simulink model "watertankLSTM"  (R2026a)
settings: Solver=ode45  StopTime=Tf  EnableMultiTasking=on
values from neighbouring files (symbols this model uses):
  Ts = 1    [DA2_main.m]    (also in LSTMController.m; TunePIControllerWithReinforcementLearningExample.m; build_compare_model.m)
undefined symbols (not defined in the file or in its folder): DiscIntNeverNeededParam
libraries: simulink x1
settings Model: Creator=The MathWorks, Inc.  LastModifiedBy=Dharu
settings DataIOCC: SignalLoggingName=logsOut
settings OptimizationCC: InitFltsAndDblsToZero=on
settings DebuggingCC: SaveWithParameterizedLinksMsg=none  SignalResolutionControl=TryResolveAllWithWarning  MultiTaskDSMMsg=warning
settings HardwareCC: ProdHWDeviceType=Specified
settings GRTTargetCC: TargetFcnLib=ansi_tfl_tmw.mat  CombineOutputUpdateFcns=off  GRTInterface=on

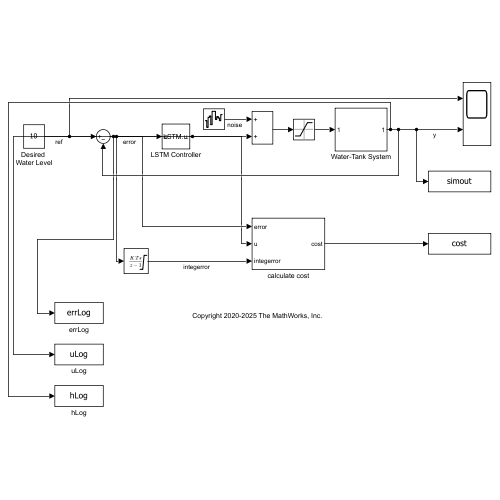
[thumbnail: Simulink's stored preview of the top-level diagram]
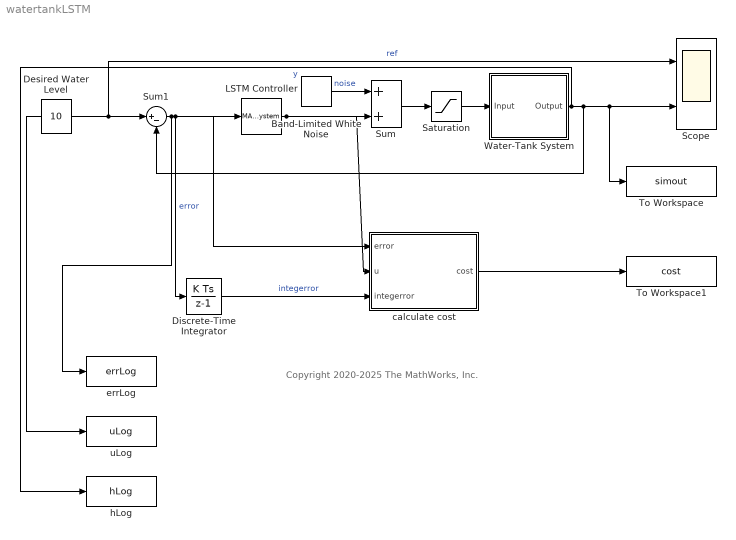
== system watertankLSTM ==
  note: Copyright 2020-2025 The MathWorks, Inc.
  Band-Limited White Noise : simulink/Sources/Band-Limited White Noise  Cov=0.01  Ts=Ts  seed=[23341]
  Desired Water Level : Constant  Value=10
  Discrete-Time Integrator : DiscreteIntegrator  gainval=1  SampleTime=Ts  LimitOutput=on  UpperSaturationLimit=100  LowerSaturationLimit=-100  ICPrevOutput=DiscIntNeverNeededParam  ICPrevScaledInput=DiscIntNeverNeededParam
  LSTM Controller : MATLABSystem  System=LSTMController  NetFile=lstmController.mat  Ts=Ts
      mask Type: LSTMController
  Saturation : Saturate  UpperLimit=12  LowerLimit=0
  Scope : Scope  NumInputPorts=2
      settings: ActiveDisplayYMinimum=-8.8693854504523131  ActiveDisplayYMaximum=18.205080928572428
  Sum : Sum
  Sum1 : Sum  Inputs=|+-  SaturateOnIntegerOverflow=on
  To Workspace : ToWorkspace  VariableName=simout  SaveFormat=Timeseries  SampleTime=-1
  To Workspace1 : ToWorkspace  VariableName=cost  SaveFormat=Timeseries  SampleTime=-1
  Water-Tank System : Subsystem
  calculate cost : Subsystem
  errLog : ToWorkspace  VariableName=errLog  SaveFormat=Timeseries  SampleTime=Ts
  hLog : ToWorkspace  VariableName=hLog  SaveFormat=Timeseries  SampleTime=Ts
  uLog : ToWorkspace  VariableName=uLog  SaveFormat=Timeseries  SampleTime=Ts
  wires:
  Desired Water Level/1 -> Scope/1, Sum1/1  "ref"
  Sum1/1 -> Discrete-Time Integrator/1, calculate cost/1(error), errLog/1, LSTM Controller/1  "error"
  Water-Tank System/1(Output) -> To Workspace/1, Scope/2, Sum1/2, hLog/1  "y"
  Sum/1 -> Saturation/1
  Band-Limited White Noise/1 -> Sum/1  "noise"
  calculate cost/1(cost) -> To Workspace1/1
  Saturation/1 -> Water-Tank System/1(Input)
  Discrete-Time Integrator/1 -> calculate cost/3(integerror)  "integerror"
  LSTM Controller/1 -> calculate cost/2(u), Sum/2, uLog/1

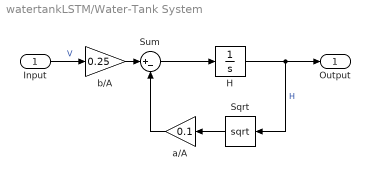
== system watertankLSTM/Water-Tank System ==
  Input : Inport
  H : Integrator  InitialCondition=1  LimitOutput=on  LowerSaturationLimit=0
  Sqrt : Sqrt  OutputSignalType=real
  Sum : Sum  Inputs=|+-  SaturateOnIntegerOverflow=on
  a/A : Gain  Gain=0.1  SaturateOnIntegerOverflow=on  OutDataTypeStr=Inherit: Same as input  ParamDataTypeStr=Inherit: Same as input
  b/A : Gain  Gain=0.25  SaturateOnIntegerOverflow=on  OutDataTypeStr=Inherit: Same as input  ParamDataTypeStr=Inherit: Same as input
  Output : Outport  VectorParamsAs1DForOutWhenUnconnected=off
  wires:
  b/A/1 -> Sum/1
  Sum/1 -> H/1
  H/1 -> Sqrt/1, Output/1  "H"
  Sqrt/1 -> a/A/1
  a/A/1 -> Sum/2
  Input/1 -> b/A/1  "V"

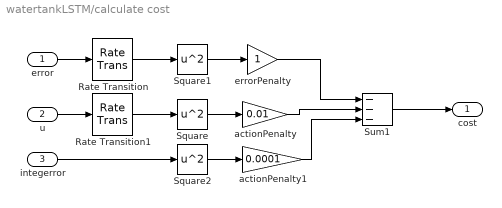
== system watertankLSTM/calculate cost ==
  error : Inport
  u : Inport  Port=2
  integerror : Inport  Port=3
  Rate Transition : RateTransition  OutPortSampleTime=Ts
  Rate Transition1 : RateTransition  OutPortSampleTime=Ts
  Square : Math  Operator=square
  Square1 : Math  Operator=square
  Square2 : Math  Operator=square
  Sum1 : Sum  Inputs=---  OutDataTypeStr=double
  actionPenalty : Gain  Gain=0.01
  actionPenalty1 : Gain  Gain=0.0001
  errorPenalty : Gain
  cost : Outport  VectorParamsAs1DForOutWhenUnconnected=off
  wires:
  Square1/1 -> errorPenalty/1
  errorPenalty/1 -> Sum1/1
  actionPenalty/1 -> Sum1/2
  Square/1 -> actionPenalty/1
  u/1 -> Rate Transition1/1
  error/1 -> Rate Transition/1
  Sum1/1 -> cost/1
  Rate Transition/1 -> Square1/1
  Rate Transition1/1 -> Square/1
  integerror/1 -> Square2/1
  actionPenalty1/1 -> Sum1/3
  Square2/1 -> actionPenalty1/1
